simulink model "Altitude"  (R2016a)
settings: Solver=ode2  StartTime=0.0  StopTime=10.0  FixedStep=sample_time  RelTol=1e-3
InitFcn:
  | Parameters_quadrotor
  | Parameters_controllers
values from neighbouring files (symbols this model uses):
  ALT_N = 30    [test.m]
  KB_H = sqrt(KD_H/KI_H)    [test.m]
  KD_H = 9    [test.m]
  KI_H = 1    [test.m]
  KP_H = 9    [test.m]
undefined symbols (not defined in the file or in its folder): MAX_DELTA_THRUST, MIN_DELTA_THRUST
libraries: simulink x1
settings Model: Creator=pela  LastModifiedBy=Mattia
settings DataIOCC: LimitDataPoints=on  SaveFormat=Array
settings DebuggingCC: AllowSymbolicDim=off
settings HardwareCC: ProdBitPerPointer=32  ProdLargestAtomicInteger=Long  ProdLargestAtomicFloat=Double  ProdIntDivRoundTo=Undefined  ProdWordSize=32  ProdHWDeviceType=ARM Compatible->ARM Cortex
settings ModelReferenceCC: PropagateSignalLabelsOutOfModel=off
settings RTWCC: GenCodeOnly=on  GenerateReport=on  BuildConfiguration=Faster Runs  LaunchReport=on  TargetLang=C++
settings GRTTargetCC: MatFileLogging=off  MultiInstanceERTCode=on  CodeInterfacePackaging=C++ class  SupportNonFinite=off
settings ConfigComp: CovModelRefEnable=Off

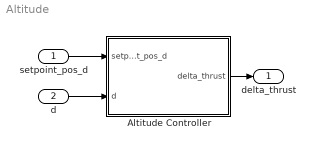
== system Altitude ==
  setpoint_pos_d : Inport
  d : Inport  Port=2
  Altitude Controller : Subsystem
  delta_thrust : Outport
  wires:
  setpoint_pos_d/1 -> Altitude Controller/1(setpoint_pos_d)
  d/1 -> Altitude Controller/2(d)
  Altitude Controller/1(delta_thrust) -> delta_thrust/1

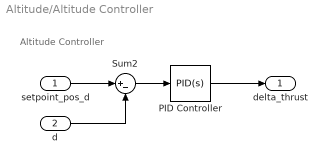
== system Altitude/Altitude Controller ==
  note: Altitude Controller
  setpoint_pos_d : Inport
  d : Inport  Port=2
  PID Controller : simulink/Continuous/PID Controller  Controller=PID  TimeDomain=Continuous-time  SampleTime=-1  IntegratorMethod=Forward Euler  FilterMethod=Trapezoidal  Form=Parallel  UseFilter=on  ControllerParametersSource=internal  P=KP_H  I=KI_H  D=KD_H  N=ALT_N  InitialConditionSource=internal  InitialConditionForIntegrator=0  InitialConditionForFilter=0  ExternalReset=none  LimitOutput=on  UpperSaturationLimit=MAX_DELTA_THRUST  LowerSaturationLimit=MIN_DELTA_THRUST  LinearizeAsGain=on  AntiWindupMode=back-calculation  Kb=KB_H  TrackingMode=off  Kt=1  PParamMin=[]  PParamMax=[]  IParamMin=[]  IParamMax=[]  DParamMin=[]  DParamMax=[]  NParamMin=[]  NParamMax=[]  KbParamMin=[]  KbParamMax=[]  KtParamMin=[]  KtParamMax=[]  POutMin=[]  POutMax=[]  IOutMin=[]  IOutMax=[]  DOutMin=[]  DOutMax=[]  NOutMin=[]  NOutMax=[]  KbOutMin=[]  KbOutMax=[]  KtOutMin=[]  KtOutMax=[]  IntegratorOutMin=[]  IntegratorOutMax=[]  FilterOutMin=[]  FilterOutMax=[]  SumOutMin=[]  SumOutMax=[]  SumI1OutMin=[]  SumI1OutMax=[]  SumI2OutMin=[]  SumI2OutMax=[]  SumI3OutMin=[]  SumI3OutMax=[]  SumDOutMin=[]  SumDOutMax=[]  SaturationOutMin=[]  SaturationOutMax=[]  IntegratorContinuousStateAttributes=''  IntegratorStateMustResolveToSignalObject=off  IntegratorRTWStateStorageClass=Auto  FilterContinuousStateAttributes=''  FilterStateMustResolveToSignalObject=off  FilterRTWStateStorageClass=Auto  DifferentiatorICPrevScaledInput=0  DifferentiatorOutMin=[]  DifferentiatorOutMax=[]
  Sum2 : Sum  Inputs=|+-
  delta_thrust : Outport
  wires:
  Sum2/1 -> PID Controller/1
  setpoint_pos_d/1 -> Sum2/1
  d/1 -> Sum2/2
  PID Controller/1 -> delta_thrust/1
